simulink model "electricUAVGCS"  (R2021b)
settings: Solver=VariableStepAuto  StartTime=0.0  StopTime=10.0  RelTol=1e-3
settings Model: Creator=mlizarra  LastModifiedBy=promero
settings SolverCC: AlgebraicLoopSolver=TrustRegion
settings DebuggingCC: SFMachineParentedDataDiag=warning
settings SFSimCC: CustomCodeUndefinedFunction=UseInterfaceOnly

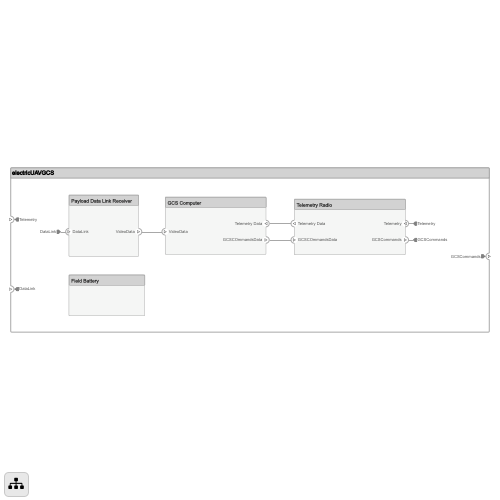
[thumbnail: Simulink's stored preview of the top-level diagram]
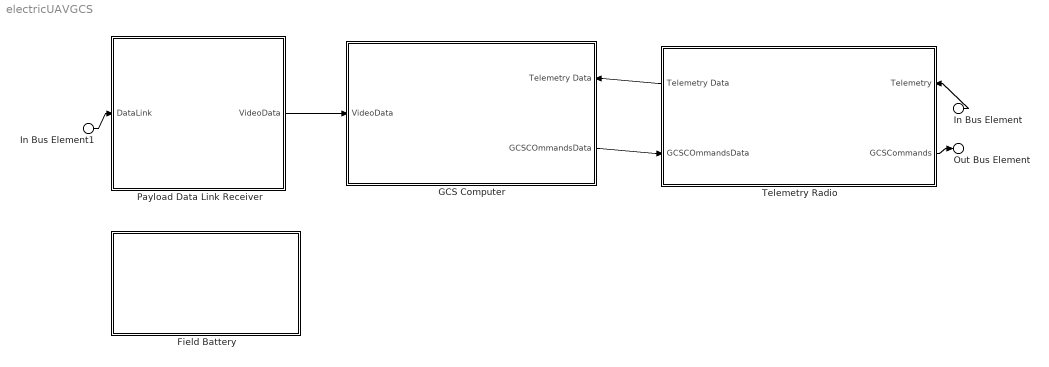
== system electricUAVGCS ==
  In Bus Element : Inport  PortName=Telemetry
  In Bus Element1 : Inport  Port=2  PortName=DataLink
  Field Battery : Subsystem
      settings: PortSchema="{\"entries\":[{\"content\":{\"headerSize\":26,\"margin\":15,\"minimumSpacing\":25,\"sides\":[{\"content\":{\"connectorIds\":[]},\"type\":\"ConnectorPlacement.EquallySpacedRectSide\",\"uuid\":\"d39ea880-6caf-4145-b7f0-b92ac95b231c\"},{\"content\":{\"connectorIds\":[],\"side\":\"RIGHT\"},\"type\":\"ConnectorPlacement.EquallySpacedRectSide\",\"uuid\":\"9a787458-5dfd-4b88-89fa-fa737c2416b2\"},{\"content\":{\"connectorIds\":[],\"side\":\"TOP\"},\"type\":\"ConnectorPlacement.EquallySpacedRectSide\",\"uuid\":\"7005747f-30ee-4956-851b-457a7a1d046d\"}]},\"type\":\"ConnectorPlacement.EquallySpacedConnector\",\"uuid\":\"a95d60af-c1bc-49cc-b537-4a2d2c040baf\"}],\"packageUris\":[\"http:\\/\\/schema.mathworks.com\\/mf0\\/Connector\\/19700101\"],\"version\":\"1.0\"}"
  GCS Computer : Subsystem
      settings: PortSchema="{\"entries\":[{\"content\":{\"headerSize\":26,\"margin\":15,\"minimumSpacing\":25,\"sides\":[{\"content\":{\"connectorIds\":[\"In1\"]},\"type\":\"ConnectorPlacement.EquallySpacedRectSide\",\"uuid\":\"d39ea880-6caf-4145-b7f0-b92ac95b231c\"},{\"content\":{\"connectorIds\":[\"In2\",\"Out1\"],\"side\":\"RIGHT\"},\"type\":\"ConnectorPlacement.EquallySpacedRectSide\",\"uuid\":\"9a787458-5dfd-4b88-89fa-fa737c2416b2\"},{\"content\":{\"connectorIds\":[],\"side\":\"TOP\"},\"type\":\"ConnectorPlacement.EquallySpacedRectSide\",\"uuid\":\"7005747f-30ee-4956-851b-457a7a1d046d\"}]},\"type\":\"ConnectorPlacement.EquallySpacedConnector\",\"uuid\":\"a95d60af-c1bc-49cc-b537-4a2d2c040baf\"}],\"packageUris\":[\"http:\\/\\/schema.mathworks.com\\/mf0\\/Connector\\/19700101\"],\"version\":\"1.0\"}"
  Payload Data Link Receiver : Subsystem
      settings: PortSchema="{\"entries\":[{\"content\":{\"headerSize\":26,\"margin\":15,\"minimumSpacing\":25,\"sides\":[{\"content\":{\"connectorIds\":[\"In1\"]},\"type\":\"ConnectorPlacement.EquallySpacedRectSide\",\"uuid\":\"d39ea880-6caf-4145-b7f0-b92ac95b231c\"},{\"content\":{\"connectorIds\":[\"Out1\"],\"side\":\"RIGHT\"},\"type\":\"ConnectorPlacement.EquallySpacedRectSide\",\"uuid\":\"9a787458-5dfd-4b88-89fa-fa737c2416b2\"},{\"content\":{\"connectorIds\":[],\"side\":\"TOP\"},\"type\":\"ConnectorPlacement.EquallySpacedRectSide\",\"uuid\":\"7005747f-30ee-4956-851b-457a7a1d046d\"}]},\"type\":\"ConnectorPlacement.EquallySpacedConnector\",\"uuid\":\"a95d60af-c1bc-49cc-b537-4a2d2c040baf\"}],\"packageUris\":[\"http:\\/\\/schema.mathworks.com\\/mf0\\/Connector\\/19700101\"],\"version\":\"1.0\"}"
  Telemetry Radio : Subsystem
      settings: PortSchema="{\"entries\":[{\"content\":{\"headerSize\":26,\"margin\":15,\"minimumSpacing\":25,\"sides\":[{\"content\":{\"connectorIds\":[\"Out1\",\"In1\"]},\"type\":\"ConnectorPlacement.EquallySpacedRectSide\",\"uuid\":\"d39ea880-6caf-4145-b7f0-b92ac95b231c\"},{\"content\":{\"connectorIds\":[\"In2\",\"Out2\"],\"side\":\"RIGHT\"},\"type\":\"ConnectorPlacement.EquallySpacedRectSide\",\"uuid\":\"9a787458-5dfd-4b88-89fa-fa737c2416b2\"},{\"content\":{\"connectorIds\":[],\"side\":\"TOP\"},\"type\":\"ConnectorPlacement.EquallySpacedRectSide\",\"uuid\":\"7005747f-30ee-4956-851b-457a7a1d046d\"}]},\"type\":\"ConnectorPlacement.EquallySpacedConnector\",\"uuid\":\"a95d60af-c1bc-49cc-b537-4a2d2c040baf\"}],\"packageUris\":[\"http:\\/\\/schema.mathworks.com\\/mf0\\/Connector\\/19700101\"],\"version\":\"1.0\"}"
  Out Bus Element : Outport  VectorParamsAs1DForOutWhenUnconnected=off  PortName=GCSCommands
  wires:
  Telemetry Radio/2(GCSCommands) -> Out Bus Element/1
  In Bus Element/1 -> Telemetry Radio/2(Telemetry)
  Telemetry Radio/1(Telemetry Data) -> GCS Computer/2(Telemetry Data)
  GCS Computer/1(GCSCOmmandsData) -> Telemetry Radio/1(GCSCOmmandsData)
  In Bus Element1/1 -> Payload Data Link Receiver/1(DataLink)
  Payload Data Link Receiver/1(VideoData) -> GCS Computer/1(VideoData)

== system electricUAVGCS/Field Battery ==

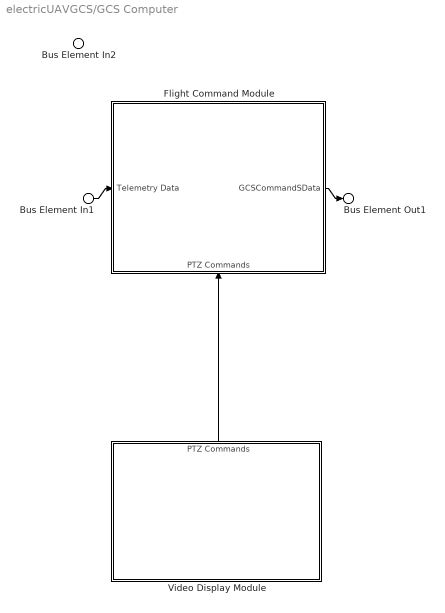
== system electricUAVGCS/GCS Computer ==
  Bus Element In2 : Inport  PortName=VideoData
  Bus Element In1 : Inport  Port=2  PortName=Telemetry Data
  Flight Command Module : Subsystem
      settings: PortSchema="{\"entries\":[{\"content\":{\"headerSize\":26,\"margin\":15,\"minimumSpacing\":25,\"sides\":[{\"content\":{\"connectorIds\":[\"In1\"]},\"type\":\"ConnectorPlacement.EquallySpacedRectSide\",\"uuid\":\"d39ea880-6caf-4145-b7f0-b92ac95b231c\"},{\"content\":{\"connectorIds\":[\"Out1\"],\"side\":\"RIGHT\"},\"type\":\"ConnectorPlacement.EquallySpacedRectSide\",\"uuid\":\"9a787458-5dfd-4b88-89fa-fa737c2416b2\"},{\"content\":{\"connectorIds\":[],\"side\":\"TOP\"},\"type\":\"ConnectorPlacement.EquallySpacedRectSide\",\"uuid\":\"7005747f-30ee-4956-851b-457a7a1d046d\"},{\"content\":{\"connectorIds\":[\"In2\"],\"side\":\"BOTTOM\"},\"type\":\"ConnectorPlacement.EquallySpacedRectSide\",\"uuid\":\"2f5eb0d8-9a60-4ca0-a751-680be560755b\"}]},\"type\":\"ConnectorPlacement.EquallySpacedConnector\",\"uuid\":\"a95d60af-c1bc-49cc-b537-4a2d2c040baf\"}],\"packageUris\":[\"http:\\/\\/schema.mathworks.com\\/mf0\\/Connector\\/19700101\"],\"version\":\"1.0\"}"
  Video Display Module : Subsystem
      settings: PortSchema="{\"entries\":[{\"content\":{\"headerSize\":26,\"margin\":15,\"minimumSpacing\":25,\"sides\":[{\"content\":{\"connectorIds\":[]},\"type\":\"ConnectorPlacement.EquallySpacedRectSide\",\"uuid\":\"d39ea880-6caf-4145-b7f0-b92ac95b231c\"},{\"content\":{\"connectorIds\":[],\"side\":\"RIGHT\"},\"type\":\"ConnectorPlacement.EquallySpacedRectSide\",\"uuid\":\"9a787458-5dfd-4b88-89fa-fa737c2416b2\"},{\"content\":{\"connectorIds\":[\"Out1\"],\"side\":\"TOP\"},\"type\":\"ConnectorPlacement.EquallySpacedRectSide\",\"uuid\":\"7005747f-30ee-4956-851b-457a7a1d046d\"}]},\"type\":\"ConnectorPlacement.EquallySpacedConnector\",\"uuid\":\"a95d60af-c1bc-49cc-b537-4a2d2c040baf\"}],\"packageUris\":[\"http:\\/\\/schema.mathworks.com\\/mf0\\/Connector\\/19700101\"],\"version\":\"1.0\"}"
  Bus Element Out1 : Outport  VectorParamsAs1DForOutWhenUnconnected=off  PortName=GCSCOmmandsData
  wires:
  Bus Element In1/1 -> Flight Command Module/1(Telemetry Data)
  Flight Command Module/1(GCSCommandSData) -> Bus Element Out1/1
  Video Display Module/1(PTZ Commands) -> Flight Command Module/2(PTZ Commands)

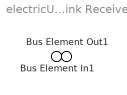
== system electricUAVGCS/Payload Data Link Receiver ==
  Bus Element In1 : Inport  PortName=DataLink
  Bus Element Out1 : Outport  VectorParamsAs1DForOutWhenUnconnected=off  PortName=VideoData
  wires:
  Bus Element In1/1 -> Bus Element Out1/1

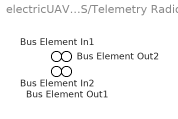
== system electricUAVGCS/Telemetry Radio ==
  Bus Element In2 : Inport  PortName=GCSCOmmandsData
  Bus Element In1 : Inport  Port=2  PortName=Telemetry
  Bus Element Out2 : Outport  VectorParamsAs1DForOutWhenUnconnected=off  PortName=Telemetry Data
  Bus Element Out1 : Outport  Port=2  VectorParamsAs1DForOutWhenUnconnected=off  PortName=GCSCommands
  wires:
  Bus Element In1/1 -> Bus Element Out2/1
  Bus Element In2/1 -> Bus Element Out1/1

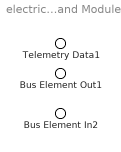
== system electricUAVGCS/GCS Computer/Flight Command Module ==
  Telemetry Data1 : Inport  PortName=Telemetry Data
  Bus Element In2 : Inport  Port=2  PortName=PTZ Commands
  Bus Element Out1 : Outport  VectorParamsAs1DForOutWhenUnconnected=off  PortName=GCSCommandSData

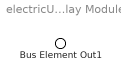
== system electricUAVGCS/GCS Computer/Video Display Module ==
  Bus Element Out1 : Outport  VectorParamsAs1DForOutWhenUnconnected=off  PortName=PTZ Commands
